simulink model "testingSOGI"  (R2023a)
settings: Solver=VariableStepAuto  StartTime=0.0  StopTime=1  RelTol=1e-3
undefined symbols (not defined in the file or in its folder): magnitude
libraries: spsabctoAlphaBetaZeroLib x1
settings Model: Creator=Anikait  LastModifiedBy=Anikait

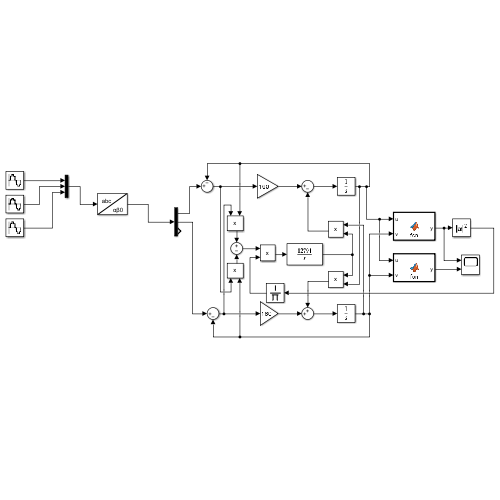
[thumbnail: Simulink's stored preview of the top-level diagram]
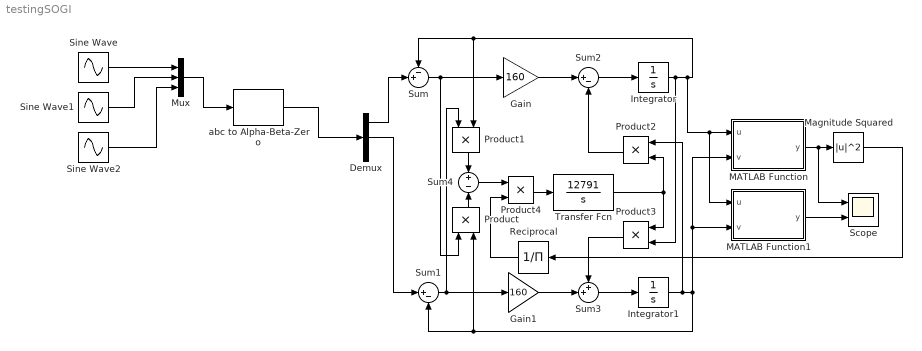
== system testingSOGI ==
  Demux : Demux  Outputs=3
  Gain : Gain  Gain=160
  Gain1 : Gain  Gain=160
  Integrator : Integrator  InitialCondition=1
  Integrator1 : Integrator  InitialCondition=1
  MATLAB Function : MATLAB Function  TreatAsAtomicUnit=on
  MATLAB Function1 : MATLAB Function  TreatAsAtomicUnit=on
  Magnitude Squared : Math  Operator=magnitude^2
  Mux : Mux  Inputs=3
  Product{,1..4} (5 alike) : Product
  Reciprocal : Product  Inputs=/  RndMeth=Zero  SaturateOnIntegerOverflow=on
  Scope : Scope  NumInputPorts=2
  Sine Wave : Sin  Amplitude=311  Frequency=2*pi*50  SampleTime=1/10000
  Sine Wave1 : Sin  Amplitude=311  Frequency=2*pi*50  Phase=2*pi/3  SampleTime=1/10000
  Sine Wave2 : Sin  Amplitude=311  Frequency=2*pi*50  Phase=4*pi/3  SampleTime=1/10000
  Sum : Sum  Inputs=-+|
  Sum1 : Sum  Inputs=|+-
  Sum2 : Sum  Inputs=|+-
  Sum3 : Sum  Inputs=++|
  Sum4 : Sum  Inputs=+-
  Transfer Fcn : TransferFcn  Numerator=[12791]  Denominator=[1 0]
  abc to Alpha-Beta-Zero : spsabctoAlphaBetaZeroLib/abc to Alpha-Beta-Zero
  wires:
  Sine Wave/1 -> Mux/1
  Sine Wave1/1 -> Mux/2
  Sine Wave2/1 -> Mux/3
  Mux/1 -> abc to Alpha-Beta-Zero/1
  abc to Alpha-Beta-Zero/1 -> Demux/1
  Demux/2 -> Sum1/1
  Sum/1 -> Product/1, Gain/1
  Sum1/1 -> Product1/1, Gain1/1
  Gain/1 -> Sum2/1
  Gain1/1 -> Sum3/2
  Demux/1 -> Sum/2
  Sum2/1 -> Integrator/1
  Sum3/1 -> Integrator1/1
  Integrator1/1 -> Product2/1, MATLAB Function1/2(v), MATLAB Function/2(v), Product/2, Sum1/2
  Integrator/1 -> Product3/2, MATLAB Function1/1(u), MATLAB Function/1(u), Product1/2, Sum/1
  Product1/1 -> Sum4/1
  Product/1 -> Sum4/2
  Sum4/1 -> Product4/1
  Product4/1 -> Transfer Fcn/1
  Transfer Fcn/1 -> Product3/1, Product2/2
  Product2/1 -> Sum2/2
  Product3/1 -> Sum3/1
  MATLAB Function/1(y) -> Scope/1, Magnitude Squared/1
  MATLAB Function1/1(y) -> Scope/2
  Magnitude Squared/1 -> Reciprocal/1
  Reciprocal/1 -> Product4/2

== matlab function testingSOGI/MATLAB Function ==
  data: u input; y output; v input
function y = fcn(u,v)

y = sqrt((u^2)+(v^2));

== matlab function testingSOGI/MATLAB Function1 ==
  data: u input; y output; v input
function y = fcn(u,v)

y = atand(v/u);
